simulink model "SP_nonlinear_LQR"  (R2016b)
settings: Solver=ode4  StartTime=0.0  StopTime=100  FixedStep=0.001  RelTol=1e-3
values from neighbouring files (symbols this model uses):
  K = lqr(P_sp,Q,R)    [SP_LQG_controller_design.m]
  Ke_sp = K_bar(:,1)    [SP_LQG_controller_design.m]    (also in controller_parameter.mat = -14.1421356237)
  Kx_sp = K_bar(:,2:end)    [SP_LQG_controller_design.m]    (also in controller_parameter.mat = [-9.4028503548 -29.2130812278])
undefined symbols (not defined in the file or in its folder): An, Aqw, Asp1, Bn, Bqw, Bsp1, Cn, Cqw, Csp1, Kn, lin_sys, Nu, Nu_inv, Nx, Ny, op
libraries: aerolibatmos2 x10, aerolib3dof2 x1, aerolib6dof2 x1, aerolibasang x1
(part 7 of 7)

== matlab function SP_nonlinear_LQR/Subsystem/sefl_built_model/Aero_coefficient/Aerodynamic coefficient ==
  data: vt input; alpha input; q input; cxt output; el input; czt output; cmt output; cbar input; xcgr input; xcg input
function [cxt,czt,cmt]=fcn(vt,alpha,q,el,cbar,xcgr,xcg)
%% ---- Look-up tables and component biuldup ------------
beta=0;
rtod = 180 / pi;
alpha=alpha*rtod;
beta=beta*rtod;
% el=el*rtod;
% ail=ail*rtod;
% rdr=rdr*rtod;
cxt = cx ( alpha, el );
%cyt = cy ( beta, ail, rdr );
czt = cz ( alpha, beta, el );
%dail = ail / 20.0;
%drdr = rdr / 30.0;
%dlda_value = dlda( alpha, beta );
%dldr_value = dldr( alpha, beta );
%clt = cl( alpha, beta ) + dlda_value * dail + dldr_value * drdr;
cmt = cm( alpha, el );
%dnda_value = dnda( alpha, beta );
%dndr_value = dndr( alpha, beta );
%cnt = cn( alpha, beta ) + dnda_value * dail + dndr_value * drdr;

%% ---- Add damping derivatives ------------
tvt = 0.5 / vt;
%b2v = b * tvt;
cq = cbar * q * tvt;
d = damping( alpha );
cxt = cxt + cq * d(1);
%cyt = cyt + b2v * ( d(2) * r + d(3) * p );
czt = czt + cq * d(4);
%clt = clt + b2v * ( d(5) * r + d(6) * p );
cmt = cmt + cq * d(7) + czt * ( xcgr - xcg );
%cnt = cnt + b2v * ( d(8)* r + d(9) * p ) - cyt * ( xcgr - xcg ) * cbar / b;

function dlda_value = dlda ( alpha, beta )

A = [ -.041  -.052  -.053  -.056  -.050  -.056  -.082  -.059  -.042  -.038  -.027  -.017;
      -.041  -.053  -.053  -.053  -.050  -.051  -.066  -.043  -.038  -.027  -.023  -.016;
      -.042  -.053  -.052  -.051  -.049  -.049  -.043  -.035  -.026  -.016  -.018  -.014;
      -.040  -.052  -.051  -.052  -.048  -.048  -.042  -.037  -.031  -.026  -.017  -.012;
      -.043  -.049  -.048  -.049  -.043  -.042  -.042  -.036  -.025  -.021  -.016  -.011;
      -.044  -.048  -.048  -.047  -.042  -.041  -.020  -.028  -.013  -.014  -.011  -.010;
      -.043  -.049  -.047  -.045  -.042  -.037  -.003  -.013  -.010  -.003  -.007  -.008 ];
A = A';  
row = 3;
col = 4;

s = 0.2 * alpha;
k = fix ( s );
if ( k <= -2 )
    k = -1;
end
if ( k >= 9 )
    k = 8;
end
da = s -  k ;
l = k + fix ( sign ( da ) * 1.1 );
%%%%%%%%%%%%%%%%%%%%%%%%%%%%%%%%%%
% added as boundary condition
if l < -2
    l = -2;
elseif l > 9
        l = 9;
end
%%%%%%%%%%%%%%%%%%%%%%%%%%%%%%%%%%
s = 0.1 * beta;
m = fix ( s );
if ( m <= -3 )
   m = -2;
end
if ( m >= 3)
   m = 2;
end
db = s -  m ;
n = m + fix ( sign ( db ) * 1.1 );
%%%%%%%%%%%%%%%%%%%%%%%%%%%%%%%%%%
% added as boundary condition
if n < -3
    n = -3;
elseif n > 3
        n = 3;
end
%%%%%%%%%%%%%%%%%%%%%%%%%%%%%%%%%%
%  disp('k+row'); k+row
%  disp('m+col'); m+col
%  disp('n+col'); n+col
%  disp('l+row'); l+row
t = A( k+row, m+col );
u = A( k+row, n+col );
v = t + abs( da ) * ( A( l+row, m+col ) - t );
w = u + abs( da ) * ( A( l+row, n+col ) - u );
dlda_value = v + ( w - v ) * abs( db );

function dldr_value = dldr ( alpha, beta )

A = [ .005  .017  .014  .010  -.005  .009  .019  .005   .000  -.005  -.011  .008;
      .007  .016  .014  .014   .013  .009  .012  .005   .000   .004   .009  .007;
      .013  .013  .011  .012   .011  .009  .008  .005   .000   .005   .003  .005;
      .018  .015  .015  .014   .014  .014  .014  .015   .013   .011   .006  .001;
      .015  .014  .013  .013   .012  .011  .011  .010   .008   .008   .007  .003;
      .021  .011  .010  .011   .010  .009  .008  .010   .006   .005   .000  .001;
      .023  .010  .011  .011   .011  .010  .008  .010   .006   .014   .020  .000 ];
A = A';  
row = 3;
col = 4;

s = 0.2 * alpha;
k = fix ( s );
if ( k <= -2 )
    k = -1;
end
if ( k >= 9 )
    k = 8;
end
da = s -  k ;
l = k + fix ( sign ( da ) * 1.1 );
%%%%%%%%%%%%%%%%%%%%%%%%%%%%%%%%%%
% added as boundary condition
if l < -2
    l = -2;
elseif l > 9
        l = 9;
end
%%%%%%%%%%%%%%%%%%%%%%%%%%%%%%%%%%
s = 0.1 * beta;
m = fix ( s );
if ( m <= -3 )
   m = -2;
end
if ( m >= 3)
   m = 2;
end
db = s -  m ;
n = m + fix ( sign ( db ) * 1.1 );
%%%%%%%%%%%%%%%%%%%%%%%%%%%%%%%%%%
% added as boundary condition
if n < -3
    n = -3;
elseif n > 3
        n = 3;
end
%%%%%%%%%%%%%%%%%%%%%%%%%%%%%%%%%%
t = A( k+row, m+col );
u = A( k+row, n+col );
v = t + abs( da ) * ( A( l+row, m+col ) - t );
w = u + abs( da ) * ( A( l+row, n+col ) - u );
dldr_value = v + ( w - v ) * abs( db );

function dnda_value = dnda ( alpha, beta )

A = [  .001  -.027  -.017  -.013  -.012  -.016   .001   .017   .011  .017   .008  .016
       .002  -.014  -.016  -.016  -.014  -.019  -.021   .002   .012  .016   .015  .011
      -.006  -.008  -.006  -.006  -.005  -.008  -.005   .007   .004  .007   .006  .006
      -.011  -.011  -.010  -.009  -.008  -.006   .000   .004   .007  .010   .004  .010
      -.015  -.015  -.014  -.012  -.011  -.008  -.002   .002   .006  .012   .011  .011
      -.024  -.010  -.004  -.002  -.001   .003   .014   .006  -.001  .004   .004  .006
      -.022   .002  -.003  -.005  -.003  -.001  -.009  -.009  -.001  .003  -.002  .001  ];
A = A';  
row = 3;
col = 4;

s = 0.2 * alpha;
k = fix ( s );
if ( k <= -2 )
    k = -1;
end
if ( k >= 9 )
    k = 8;
end
da = s -  k ;
l = k + fix ( sign ( da ) * 1.1 );
%%%%%%%%%%%%%%%%%%%%%%%%%%%%%%%%%%
% added as boundary condition
if l < -2
    l = -2;
elseif l > 9
        l = 9;
end
%%%%%%%%%%%%%%%%%%%%%%%%%%%%%%%%%%
s = 0.1 * beta;
m = fix ( s );
if ( m <= -3 )
   m = -2;
end
if ( m >= 3)
   m = 2;
end
db = s -  m ;
n = m + fix ( sign ( db ) * 1.1 );
%%%%%%%%%%%%%%%%%%%%%%%%%%%%%%%%%%
% added as boundary condition
if n < -3
    n = -3;
elseif n > 3
        n = 3;
end
%%%%%%%%%%%%%%%%%%%%%%%%%%%%%%%%%%
t = A( k+row, m+col );
u = A( k+row, n+col );
v = t + abs( da ) * ( A( l+row, m+col ) - t );
w = u + abs( da ) * ( A( l+row, n+col ) - u );
dnda_value = v + ( w - v ) * abs( db );

function dndr_value = dndr ( alpha, beta )

A = [ -.018  -.052  -.052  -.052  -.054  -.049  -.059  -.051  -.030  -.037  -.026  -.013;
      -.028  -.051  -.043  -.046  -.045  -.049  -.057  -.052  -.030  -.033  -.030  -.008;
      -.037  -.041  -.038  -.040  -.040  -.038  -.037  -.030  -.027  -.024  -.019  -.013; 
      -.048  -.045  -.045  -.045  -.044  -.045  -.047  -.048  -.049  -.045  -.033  -.016;
      -.043  -.044  -.041  -.041  -.040  -.038  -.034  -.035  -.035  -.029  -.022  -.009;
      -.052  -.034  -.036  -.036  -.035  -.028  -.024  -.023  -.020  -.016  -.010  -.014;
      -.062  -.034  -.027  -.028  -.027  -.027  -.023  -.023  -.019  -.009  -.025  -.010 ];
A = A';  
row = 3;
col = 4;

s = 0.2 * alpha;
k = fix ( s );
if ( k <= -2 )
    k = -1;
end
if ( k >= 9 )
    k = 8;
end
da = s -  k ;
l = k + fix ( sign ( da ) * 1.1 );
%%%%%%%%%%%%%%%%%%%%%%%%%%%%%%%%%%
% added as boundary condition
if l < -2
    l = -2;
elseif l > 9
        l = 9;
end
%%%%%%%%%%%%%%%%%%%%%%%%%%%%%%%%%%
s = 0.1 * beta;
m = fix ( s );
if ( m <= -3 )
   m = -2;
end
if ( m >= 3)
   m = 2;
end
db = s -  m ;
n = m + fix ( sign ( db ) * 1.1 );
%%%%%%%%%%%%%%%%%%%%%%%%%%%%%%%%%%
% added as boundary condition
if n < -3
    n = -3;
elseif n > 3
        n = 3;
end
%%%%%%%%%%%%%%%%%%%%%%%%%%%%%%%%%%
t = A( k+row, m+col );
u = A( k+row, n+col );
v = t + abs( da ) * ( A( l+row, m+col ) - t );
w = u + abs( da ) * ( A( l+row, n+col ) - u );
dndr_value = v + ( w - v ) * abs( db );

function cx_value = cx( alpha, el )

A = [ -0.099  -0.081  -0.081  -0.063  -0.025  0.044  0.097  0.113  0.145  0.167  0.174  0.166;
      -0.048  -0.038  -0.040  -0.021   0.016  0.083  0.127  0.137  0.162  0.177  0.179  0.167;
      -0.022  -0.020  -0.021  -0.004   0.032  0.094  0.128  0.130  0.154  0.161  0.155  0.138;
      -0.040  -0.038  -0.039  -0.025   0.006  0.062  0.087  0.085  0.100  0.110  0.104  0.091;
      -0.083  -0.073  -0.076  -0.072  -0.046  0.012  0.024  0.025  0.043  0.053  0.047  0.040 ];
A = A';  
row = 3;
col = 3;

s = 0.2 * alpha;
k = fix ( s );
if ( k <= -2 )
    k = -1;
end
if ( k >= 9 )
    k = 8;
end
da = s - k;
l = k + fix ( sign ( da ) * 1.1 );
%%%%%%%%%%%%%%%%%%%%%%%%%%%%%%%%%%
% added as boundary condition
if l < -2
    l = -2;
elseif l > 9
        l = 9;
end
%%%%%%%%%%%%%%%%%%%%%%%%%%%%%%%%%%
s = el / 12.0;
m = fix ( s );
if ( m <= -2 )
   m = -1;
end
if ( m >= 2)
   m = 1;
end
de = s - m;
n = m + fix ( sign ( de ) * 1.1 );
%%%%%%%%%%%%%%%%%%%%%%%%%%%%%%%%%%
% added as boundary condition
if n < -2
    n = -2;
elseif n > 2
        n = 2;
end
%%%%%%%%%%%%%%%%%%%%%%%%%%%%%%%%%%
t = A( k+row, m+col );
u = A( k+row, n+col );
v = t + abs( da ) * ( A( l+row, m+col ) - t );
w = u + abs( da ) * ( A( l+row, n+col ) - u );
cx_value = v + ( w - v ) * abs( de );

function cy_value = cy( beta, ail, rdr )

cy_value = -0.02 * beta + 0.021 * ( ail / 20.0 )+...
           0.086 * ( rdr / 30.0 );
       
function cz_value = cz( alpha, beta, el )

A = [ 0.770  0.241  -0.100  -0.416  -0.731  -1.053  -1.366  -1.646  -1.917  -2.120  -2.248  -2.229 ];
A = A';  
row = 3;

s = 0.2 * alpha;
k = fix ( s );
if ( k <= -2 )
    k = -1;
end
if ( k >= 9 )
    k = 8;
end
da = s - k;
l = k + fix ( sign ( da ) * 1.1 );
%%%%%%%%%%%%%%%%%%%%%%%%%%%%%%%%%%
% added as boundary condition
if l < -2
    l = -2;
elseif l > 9
        l = 9;
end
%%%%%%%%%%%%%%%%%%%%%%%%%%%%%%%%%%
s = A( k+row ) + abs( da ) * ( A( l+row ) - A( k+row ) );
cz_value = s * ( 1 - ( beta / 57.3 ) ^ 2 ) - 0.19 * ( el / 25.0 );

function cl_value = cl( alpha, beta )

A = [  .0     .0     .0     .0     .0     .0     .0     .0     .0     .0     .0     .0  ;
      -.001  -.004  -.008  -.012  -.016  -.022  -.022  -.021  -.015  -.008  -.013  -.015;
      -.003  -.009  -.017  -.024  -.030  -.041  -.045  -.040  -.016  -.002  -.010  -.019;
      -.001  -.010  -.020  -.030  -.039  -.054  -.057  -.054  -.023  -.006  -.014  -.027;
       .000  -.010  -.022  -.034  -.047  -.060  -.069  -.067  -.033  -.036  -.035  -.035;
       .007  -.010  -.023  -.034  -.049  -.063  -.081  -.079  -.060  -.058  -.062  -.059;
       .009  -.011  -.023  -.037  -.050  -.068  -.089  -.088  -.091  -.076  -.077  -.076 ];
A = A'; 
row = 3;
col = 1;

s = 0.2 * alpha;
k = fix ( s );
if ( k <= -2 )
    k = -1;
end
if ( k >= 9 )
    k = 8;
end
da = s - k;
l = k + fix( sign ( da ) * 1.1 );
%%%%%%%%%%%%%%%%%%%%%%%%%%%%%%%%%%
% added as boundary condition
if l < -2
    l = -2;
elseif l > 9
        l = 9;
end
%%%%%%%%%%%%%%%%%%%%%%%%%%%%%%%%%%
s = 0.2 * abs( beta );
m = fix ( s );
if ( m == 0 )
   m = 1;
end
if ( m >= 6)
   m = 5;
end
db = s - m;
n = m + fix ( sign ( db ) * 1.1 );
%%%%%%%%%%%%%%%%%%%%%%%%%%%%%%%%%%
% added as boundary condition
if n < 0
    n = 0;
elseif n > 6
        n = 6;
end
%%%%%%%%%%%%%%%%%%%%%%%%%%%%%%%%%%
t = A( k+row, m+col );
u = A( k+row, n+col );
v = t + abs( da ) * ( A( l+row, m+col ) - t );
w = u + abs( da ) * ( A( l+row, n+col ) - u );
dum = v + ( w - v ) * abs( db );
cl_value = dum * sign ( beta ) * 1.0;

function cm_value = cm( alpha, el )

A = [ .205   .168   .186   .196   .213   .251   .245   .238   .252   .231   .198   .192;
      .081   .077   .107   .110   .110   .141   .127   .119   .133   .108   .081   .093;
     -.046  -.020  -.009  -.005  -.006   .010   .006  -.001   .014   .000  -.013   .032;
     -.174  -.145  -.121  -.127  -.129  -.102  -.097  -.113  -.087  -.084  -.069  -.006;
     -.259  -.202  -.184  -.193  -.199  -.150  -.160  -.167  -.104  -.076  -.041  -.005 ];
A = A';  
row = 3;
col = 3;

s = 0.2 * alpha;
k = fix ( s );
if ( k <= -2 )
    k = -1;
end
if ( k >= 9 )
    k = 8;
end
da = s - k;
l = k + fix ( sign ( da ) * 1.1 );
%%%%%%%%%%%%%%%%%%%%%%%%%%%%%%%%%%
% added as boundary condition
if l < -2
    l = -2;
elseif l > 9
        l = 9;
end
%%%%%%%%%%%%%%%%%%%%%%%%%%%%%%%%%%
s = el / 12.0;
m = fix ( s );
if ( m <= -2 )
   m = -1;
end
if ( m >= 2)
   m = 1;
end
de = s - m;
n = m + fix ( sign ( de ) * 1.1 );
%%%%%%%%%%%%%%%%%%%%%%%%%%%%%%%%%%
% added as boundary condition
if n < -2
    n = -2;
elseif n > 2
        n = 2;
end
%%%%%%%%%%%%%%%%%%%%%%%%%%%%%%%%%%
t = A( k+row, m+col );
u = A( k+row, n+col );
v = t + abs( da ) * ( A( l+row, m+col ) - t );
w = u + abs( da ) * ( A( l+row, n+col ) - u );
cm_value = v + ( w - v ) * abs( de );

function cn_value = cn( alpha, beta )

A = [ .0    .0    .0    .0    .0    .0    .0    .0    .0     .0     .0     .0  ;
      .018  .019  .018  .019  .019  .018  .013  .007  .004  -.014  -.017  -.033;
      .038  .042  .042  .042  .043  .039  .030  .017  .004  -.035  -.047  -.057;
      .056  .057  .059  .058  .058  .053  .032  .012  .002  -.046  -.071  -.073;
      .064  .077  .076  .074  .073  .057  .029  .007  .012  -.034  -.065  -.041;
      .074  .086  .093  .089  .080  .062  .049  .022  .028  -.012  -.002  -.013;
      .079  .090  .106  .106  .096  .080  .068  .030  .064   .015   .011  -.001 ];
A = A';  
row = 3;
col = 1;
  
s = 0.2 * alpha;
k = fix ( s );
if ( k <= -2 )
    k = -1;
end
if ( k >= 9 )
    k = 8;
end
da = s - k;
l = k + fix ( sign ( da ) * 1.1 );
%%%%%%%%%%%%%%%%%%%%%%%%%%%%%%%%%%
% added as boundary condition
if l < -2
    l = -2;
elseif l > 9
        l = 9;
end
%%%%%%%%%%%%%%%%%%%%%%%%%%%%%%%%%%
s = 0.2 * abs( beta );
m = fix ( s );
if ( m == 0 )
   m = 1;
end
if ( m >= 6)
   m = 5;
end
db = s - m;
n = m + fix ( sign ( db ) * 1.1 );
%%%%%%%%%%%%%%%%%%%%%%%%%%%%%%%%%%
% added as boundary condition
if n < 0
    n = 0;
elseif n > 6
        n = 6;
end
%%%%%%%%%%%%%%%%%%%%%%%%%%%%%%%%%%
t = A( k+row, m+col );
u = A( k+row, n+col );
v = t + abs( da ) * ( A( l+row, m+col ) - t );
w = u + abs( da ) * ( A( l+row, n+col ) - u );
dum = v + ( w - v ) * abs( db );
cn_value = dum * sign ( beta ) * 1.0;

function [ d ] = damping ( alpha )  

% d1 = CXq;
% d2 = CYr;
% d3 = CYp;
% d4 = CZq;
% d5 = Clr;
% d6 = Clp;
% d7 = Cmq;
% d8 = Cnr;
% d9 = Cnp;


A = [ -0.267   -0.110    0.308    1.34     2.08     2.91     2.76     2.05     1.50    1.49    1.83    1.21;
       0.882    0.852    0.876    0.958    0.962    0.974    0.819    0.483    0.590   1.21   -0.493  -1.04;
      -0.108   -0.108   -0.188    0.110    0.258    0.226    0.344    0.362    0.611   0.529   0.298  -0.227;
      -8.80    -25.8    -28.9    -31.4    -31.2    -30.7    -27.7    -28.2    -29.0   -29.8   -38.3   -35.3;
      -0.126   -0.026    0.063    0.113    0.208    0.230    0.319    0.437    0.680   0.100   0.447  -0.330;
      -0.360   -0.359   -0.443   -0.420   -0.383   -0.375   -0.329   -0.294   -0.230  -0.210  -0.120  -0.100;
      -7.21    -5.40    -5.23    -5.26    -6.11    -6.64    -5.69    -6.00    -6.20   -6.40   -6.60   -6.00;
      -0.380   -0.363   -0.378   -0.386   -0.370   -0.453   -0.550   -0.582   -0.595  -0.637  -1.02   -0.840;
       0.061    0.052    0.052   -0.012   -0.013   -0.024    0.050    0.150    0.130   0.158   0.240   0.150 ];
A = A';  
row = 3;

s = 0.2 * alpha;
k = fix ( s );
if ( k <= -2 )
    k = -1;
elseif ( k >= 9 )
    k = 8;
end
da = s - k;
l = k + fix ( sign ( da ) * 1.1 );
%%%%%%%%%%%%%%%%%%%%%%%%%%%%%%%%%%
% added as boundary condition
if l < -2
    l = -2;
elseif l > 9
        l = 9;
end
%%%%%%%%%%%%%%%%%%%%%%%%%%%%%%%%%%
d=zeros(1,9);
for ( i = 1 : 9 ) % step : i++
    d( i ) = A( k+row, i ) + abs( da ) * ( A( l+row, i ) - A( k+row, i ) );
end
d = d'; % transfer d into a column vector

== matlab function SP_nonlinear_LQR/Subsystem/sefl_built_model/Flight_dynamics/MATLAB Function ==
  data: V output; w input; u input; alpha output; w_dot input; u_dot input; alpha_dot output; V_dot output
function [V,alpha,alpha_dot,V_dot] = fcn(w,u,w_dot,u_dot)
V=400;
alpha = atan(w/u);
%V=(u^2+w^2)^0.5;
alpha_dot=(u*w_dot-w*u_dot)/V^2;
V_dot=(u*u_dot+w*w_dot)/V;

== matlab function SP_nonlinear_LQR/Subsystem/sefl_built_model/MATLAB Function2 ==
  data: W input; X output; theta input; phi input; Y output; Z output
function [X,Y,Z] = fcn(W,theta,phi)
X=-W*sin(theta);
Y=W*cos(theta)*sin(phi);
Z=W*cos(theta)*cos(phi);

== matlab function SP_nonlinear_LQR/Subsystem/sefl_built_model/dynamic head ==
  data: v input; qbar output; rho input
function qbar = fcn(v,rho)
qbar=0.5*rho*v^2;

== matlab function SP_nonlinear_LQR/Subsystem/sefl_built_model/thrust model ==
  data: pow input; thrust_value output; alt input; rmach input
function thrust_value = thrust ( pow, alt, rmach )
% A - idle
% B - military
% A - maximum

A = [  1060.0    670.0     880.0    1140.0  1500.0   1860.0; 
       635.0     425.0     690.0    1010.0  1330.0   1700.0;
        60.0     25.0      345.0     755.0  1130.0   1525.0;
      -1020.0    -710.0   -300.0     350.0   910.0   1360.0;
      -2700.0   -1900.0   -1300.0   -247.0   600.0   1100.0;
      -3600.0   -1400.0   -595.0    -342.0  -200.0    700.0 ];
A = A';  
  
B = [ 12680.0  9150.0    6200.0   3950.0   2450.0   1400.0;
      12680.0  9150.0    6313.0   4040.0   2470.0   1400.0;
      12610.0  9312.0    6610.0   4290.0   2600.0   1560.0;
      12640.0  9839.0    7090.0   4660.0   2840.0   1660.0;
      12390.0  10176.0   7750.0   5320.0   3250.0   1930.0;
      11680.0  9848.0    8050.0   6100.0   3800.0   2310.0 ];
B = B';  

C = [ 20000.0  15000.0  10800.0   7000.0   4000.0   2500.0;
      21420.0  15700.0  11225.0   7323.0   4435.0   2600.0;
      22700.0  16860.0  12250.0   8154.0   5000.0   2835.0;
      24240.0  18910.0  13760.0   9285.0   5700.0   3215.0;
      26070.0  21075.0  15975.0  11115.0   6860.0   3950.0;
      28886.0  23319.0  18300.0  13484.0   8642.0   5057.0 ];  
C = C';  

row = 1;
col = 1;

h = 0.0001 * alt;
i = fix( h );
if (i >= 5)
    i = 4;
elseif (i <= 0)
     i = 0;
end
dh = h - i;
rm = 5.0 * rmach;
%  disp('rmach'); rmach
m = fix( rm );
if ( m >= 5 )
    m = 4;
elseif (m <= 0)
     m = 0;
end
dm = rm - m;
cdh = 1.0 - dh;
%  disp('i+row'); i+row
%  disp('m+row'); m+row
s = B( i+row, m+col ) * cdh + B( i+1+row, m+col ) * dh;
t = B( i+row, m+1+col ) * cdh + B( i+1+row, m+1+col ) * dh;
tmil = s + ( t - s ) * dm;
if( pow < 50.0 )
    s = A( i+row, m+col )   * cdh + A( i+1+row, m+col ) * dh;
    t = A( i+row, m+1+col ) * cdh + A( i+1+row, m+1+col ) * dh;
    tidl = s + ( t - s ) * dm;
    thrust_value = tidl + ( tmil - tidl ) * pow *0.02;
else
    s = C( i+row, m+col )   * cdh + C( i+1+row, m+col ) * dh;
    t = C( i+row, m+1+col ) * cdh + C( i+1+row, m+1+col ) * dh;
    tmax = s + ( t - s ) * dm;
    thrust_value = tmil + ( tmax - tmil ) * ( pow - 50.0 ) * 0.02;
end
